simulink model "Evaporator_Simulink_LQI"  (R2025b)
settings: Solver=VariableStepAuto  StartTime=t0  StopTime=tfin  RelTol=1e-3
values from neighbouring files (symbols this model uses):
  K_i = K_lqi(:, 4:6)    [evaporator_LQI_structure.m]
  K_x = K_lqi(:, 1:3)    [evaporator_LQI_structure.m]
  L2_opt = xOpt(2)    [evaporator_LQI_structure.m]
  P2_opt = xOpt(1)    [evaporator_LQI_structure.m]
  u_mv_nom = u_full_nom(mv_idx)    [evaporator_LQI_structure.m]
  X2_opt = xOpt(3)    [evaporator_LQI_structure.m]
  x_nom = [L2_opt; X2_opt; P2_opt]    [evaporator_LQI_structure.m]
undefined symbols (not defined in the file or in its folder): dist
libraries: simulink x7
settings Model: Creator=maxen  LastModifiedBy=malcolmrenney

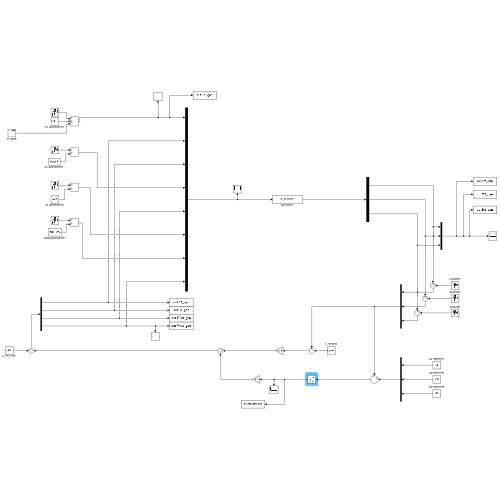
[thumbnail: Simulink's stored preview of the top-level diagram]
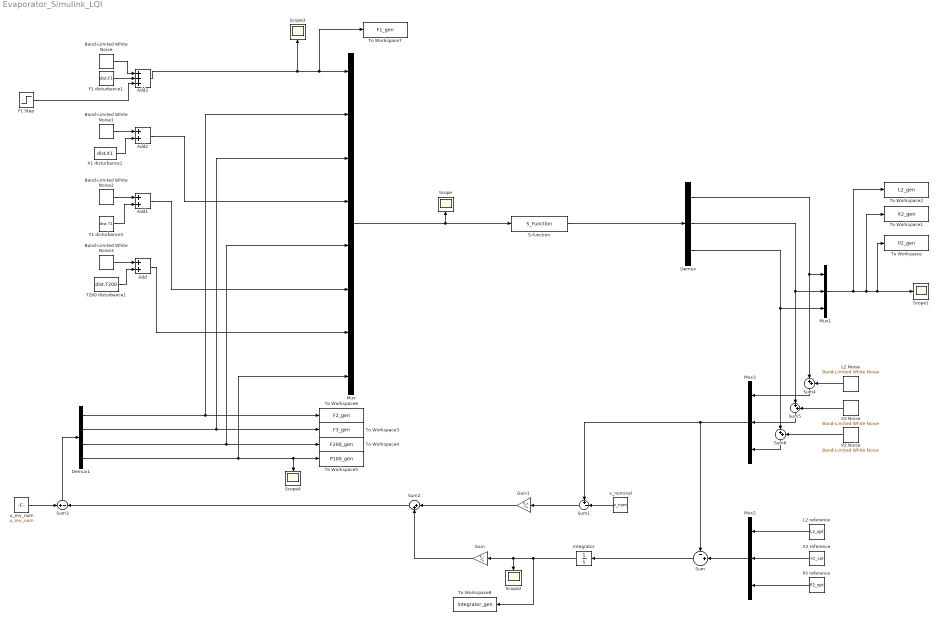
== system Evaporator_Simulink_LQI ==
  Add : Sum
  Add1 : Sum
  Add2 : Sum
  Add3 : Sum  Inputs=+++
  Band-Limited White Noise{,1..3} (4 alike) : simulink/Sources/Band-Limited White Noise  Cov=[0.1]  Ts=0.5  seed=[23341]
  Demux : Demux  Outputs=3
  Demux1 : Demux
  F1 Step : Step  Time=2000  After=2  SampleTime=0
  F1 disturbance1 : Constant  Value=dist.F1
  Gain : Gain  Gain=K_i  Multiplication=Matrix(K*u)
  Gain1 : Gain  Gain=K_x  Multiplication=Matrix(K*u)
  Integrator : Integrator  LimitOutput=on
  L2 Noise : simulink/Sources/Band-Limited White Noise  Cov=var_L  Ts=1  seed=[23341]
  L2 reference : Constant  Value=L2_opt
  Mux : Mux  Inputs=8
  Mux1 : Mux  Inputs=3
  Mux2 : Mux  Inputs=3
  Mux3 : Mux  Inputs=3
  P2 Noise : simulink/Sources/Band-Limited White Noise  Cov=var_P  Ts=1  seed=[23341]
  P2 reference : Constant  Value=P2_opt
  "S-function " : S-Function  FunctionName=S_Function  Parameters=xinit, par  SFunctionDeploymentMode=off  EnableBusSupport=off
  Scope{,1..4} (5 alike) : Scope
      Scope settings: ActiveDisplayYMinimum=-17.035908908454843  ActiveDisplayYMaximum=279.17268002477897
      Scope1 settings: ActiveDisplayYMinimum=-10.134387403024906  ActiveDisplayYMaximum=101.20948662721952
      Scope2 settings: ActiveDisplayYMinimum=-4007.6400376564029  ActiveDisplayYMaximum=646.69418647878  DataLoggingVariableName=ScopeData2
      Scope3 settings: ActiveDisplayYMinimum=7.745340223241338  ActiveDisplayYMaximum=14.169090746878569  DataLoggingVariableName=ScopeData3
      Scope4 settings: ActiveDisplayYMinimum=212.8416095314978  ActiveDisplayYMaximum=340.1833316441959  DataLoggingVariableName=ScopeData4
  Sum : Sum  Inputs=-+|
  Sum1 : Sum  Inputs=+-|
  Sum{2,4..6} (4 alike) : Sum  Inputs=|++
  Sum3 : Sum  Inputs=+|-
  T1 disturbance1 : Constant  Value=dist.T1
  T200 disturbance1 : Constant  Value=dist.T200
  To Workspace : ToWorkspace  VariableName=P2_gen  SampleTime=-1
  To Workspace1 : ToWorkspace  VariableName=X2_gen  SampleTime=-1
  To Workspace2 : ToWorkspace  VariableName=L2_gen  SampleTime=-1
  To Workspace3 : ToWorkspace  VariableName=F3_gen  SampleTime=-1
  To Workspace4 : ToWorkspace  VariableName=F200_gen  SampleTime=-1
  To Workspace5 : ToWorkspace  VariableName=P100_gen  SampleTime=-1
  To Workspace6 : ToWorkspace  VariableName=F2_gen  SampleTime=-1
  To Workspace7 : ToWorkspace  VariableName=F1_gen  SampleTime=-1
  To Workspace8 : ToWorkspace  VariableName=integrator_gen  SampleTime=-1
  X1 disturbance1 : Constant  Value=dist.X1
  X2 Noise : simulink/Sources/Band-Limited White Noise  Cov=var_X  Ts=1  seed=[23341]
  X2 reference : Constant  Value=X2_opt
  u_mv_nom : Constant  Value=u_mv_nom
  x_nominal : Constant  Value=x_nom  VectorParams1D=off
  wires:
  Mux/1 -> Scope/1, "S-function "/1
  "S-function "/1 -> Demux/1
  Mux2/1 -> Sum/2
  x_nominal/1 -> Sum1/2
  Sum1/1 -> Gain1/1
  u_mv_nom/1 -> Sum3/1
  Sum2/1 -> Sum3/2
  Gain/1 -> Sum2/2
  Demux/3 -> Sum6/1, Mux1/3
  Demux/2 -> Sum5/1, Mux1/2
  Demux/1 -> Sum4/1, Mux1/1
  Demux1/2 -> Mux/3, To Workspace3/1
  Demux1/3 -> Mux/5, To Workspace4/1
  Demux1/4 -> Mux/8, To Workspace5/1, Scope4/1
  Add1/1 -> Mux/6
  Sum/1 -> Integrator/1
  Integrator/1 -> Gain/1, Scope2/1, To Workspace8/1
  L2 Noise/1 -> Sum4/2
  X2 Noise/1 -> Sum5/2
  P2 Noise/1 -> Sum6/2
  Sum4/1 -> Mux3/1
  Sum5/1 -> Mux3/2
  Sum6/1 -> Mux3/3
  Mux3/1 -> Sum/1, Sum1/1
  Mux1/1 -> To Workspace2/1, To Workspace1/1, Scope1/1, To Workspace/1
  P2 reference/1 -> Mux2/3
  L2 reference/1 -> Mux2/1
  X2 reference/1 -> Mux2/2
  Demux1/1 -> Mux/2, To Workspace6/1
  Band-Limited White Noise2/1 -> Add1/1
  Band-Limited White Noise3/1 -> Add/1
  Band-Limited White Noise/1 -> Add3/1
  Band-Limited White Noise1/1 -> Add2/1
  T1 disturbance1/1 -> Add1/2
  X1 disturbance1/1 -> Add2/2
  F1 disturbance1/1 -> Add3/2
  T200 disturbance1/1 -> Add/2
  Add3/1 -> Mux/1, To Workspace7/1, Scope3/1
  Add2/1 -> Mux/4
  Add/1 -> Mux/7
  Sum3/1 -> Demux1/1
  Gain1/1 -> Sum2/1
  F1 Step/1 -> Add3/3
